simulink model "CoffeeReactor_task1"  (R2023b)
settings: Solver=ode4  StartTime=0.0  StopTime=simulationParameters.Tsim  FixedStep=simulationParameters.Tint  RelTol=1e-3
undefined symbols (not defined in the file): controller_parameters, myPID, ReactorModel_StateUpdate, simulationParameters
settings Model: Creator=simone  LastModifiedBy=viola
settings SolverCC: AlgebraicLoopSolver=TrustRegion
settings DataIOCC: SaveOutput=off  SignalLogging=off  DSMLogging=off  SaveTime=off  ReturnWorkspaceOutputs=off
settings DebuggingCC: UnconnectedInputMsg=warning  UnconnectedOutputMsg=warning  UnconnectedLineMsg=warning
settings ModelReferenceCC: EnableRefExpFcnMdlSchedulingChecks=on
settings RTWCC: DLArmComputeVersion=19.05

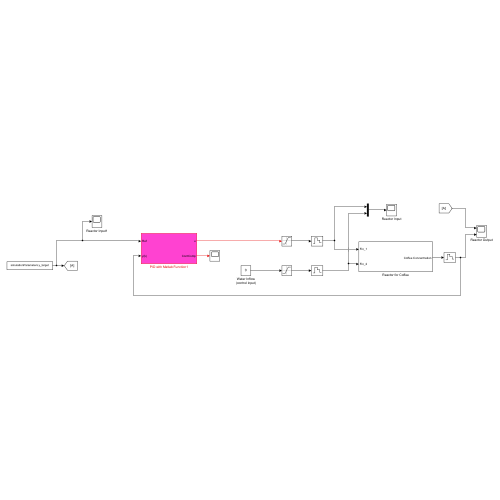
[thumbnail: Simulink's stored preview of the top-level diagram]
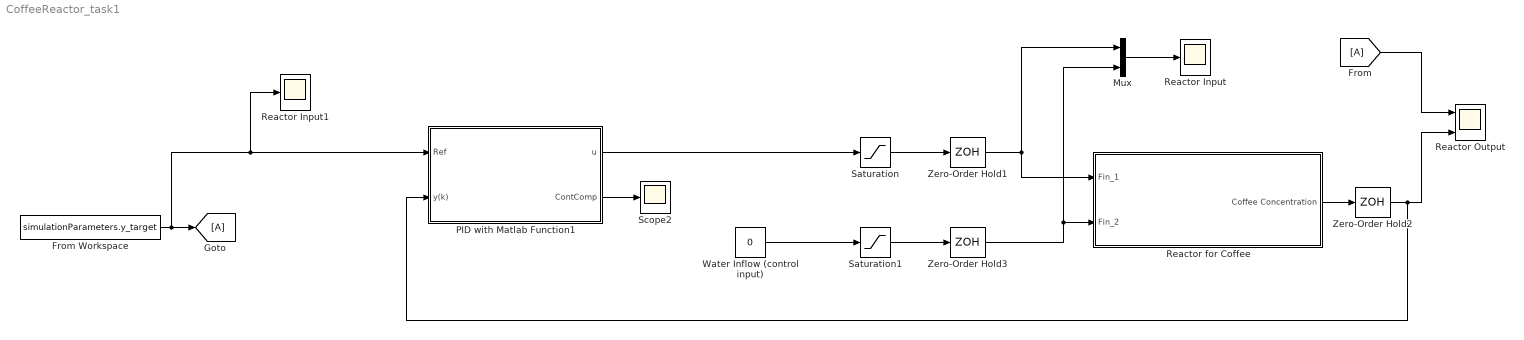
== system CoffeeReactor_task1 ==
  From : From
  From Workspace : FromWorkspace  VariableName=simulationParameters.y_target  OutputAfterFinalValue=Holding final value
  Goto : Goto
  Mux : Mux  Inputs=2
  PID with Matlab Function1 : Subsystem
  Reactor Input : Scope
  Reactor Input1 : Scope
  Reactor Output : Scope  NumInputPorts=2
  Reactor for Coffee : Subsystem
  Saturation : Saturate  UpperLimit=simulationParameters.Fin1_max  LowerLimit=simulationParameters.Fin1_min
  Saturation1 : Saturate  UpperLimit=simulationParameters.Fin2_max  LowerLimit=simulationParameters.Fin2_min
  Scope2 : Scope
  Water Inflow (control input) : Constant  Value=0
  Zero-Order Hold1 : ZeroOrderHold  SampleTime=simulationParameters.Ts
  Zero-Order Hold2 : ZeroOrderHold  SampleTime=simulationParameters.Ts
  Zero-Order Hold3 : ZeroOrderHold  SampleTime=simulationParameters.Ts
  wires:
  Reactor for Coffee/1(Coffee Concentration) -> Zero-Order Hold2/1
  Zero-Order Hold2/1 -> PID with Matlab Function1/2(y(k)), Reactor Output/2
  From/1 -> Reactor Output/1
  Mux/1 -> Reactor Input/1
  Water Inflow (control input)/1 -> Saturation1/1
  PID with Matlab Function1/1(u) -> Saturation/1
  Zero-Order Hold1/1 -> Reactor for Coffee/1(Fin_1), Mux/1
  Zero-Order Hold3/1 -> Reactor for Coffee/2(Fin_2), Mux/2
  Saturation/1 -> Zero-Order Hold1/1
  Saturation1/1 -> Zero-Order Hold3/1
  From Workspace/1 -> Reactor Input1/1, PID with Matlab Function1/1(Ref), Goto/1
  PID with Matlab Function1/2(ContComp) -> Scope2/1

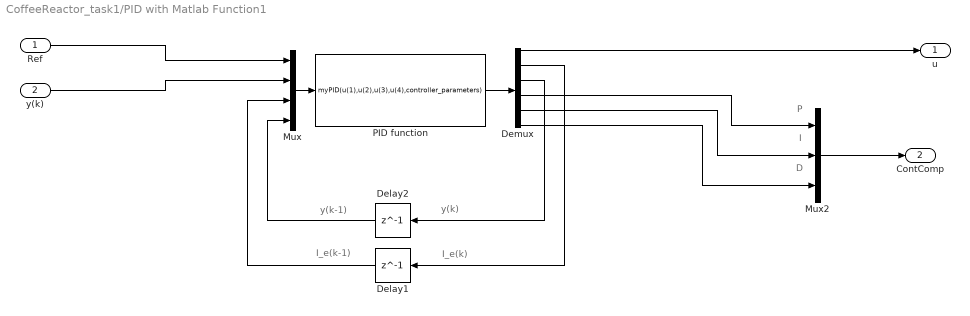
== system CoffeeReactor_task1/PID with Matlab Function1 ==
  note: y(k-1)
  note: y(k)
  note: D
  note: I
  note: P
  note: I_e(k)
  note: I_e(k-1)
  Ref : Inport
  y(k) : Inport  Port=2
  Delay1 : Delay  DelayLength=1
  Delay2 : Delay  DelayLength=1
  Demux : Demux  Outputs=6
  Mux : Mux
  Mux2 : Mux  Inputs=3
  PID function : MATLABFcn  MATLABFcn=myPID(u(1),u(2),u(3),u(4),controller_parameters)  OutputDimensions=6
  u : Outport
  ContComp : Outport  Port=2
  wires:
  Ref/1 -> Mux/1
  y(k)/1 -> Mux/2
  Mux/1 -> PID function/1
  PID function/1 -> Demux/1
  Demux/1 -> u/1
  Demux/4 -> Mux2/1
  Demux/5 -> Mux2/2
  Demux/6 -> Mux2/3
  Demux/2 -> Delay1/1
  Delay1/1 -> Mux/3
  Mux2/1 -> ContComp/1
  Delay2/1 -> Mux/4
  Demux/3 -> Delay2/1

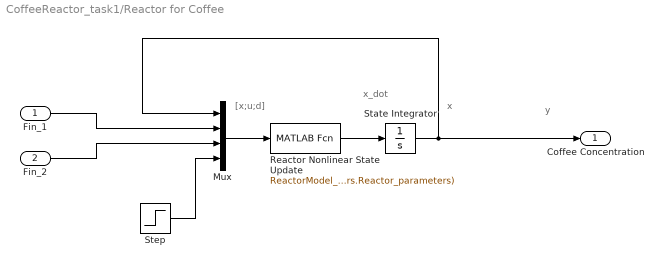
== system CoffeeReactor_task1/Reactor for Coffee ==
  note: y
  note: [x;u;d]
  note: x
  note: x_dot
  Fin_1 : Inport
  Fin_2 : Inport  Port=2
  Mux : Mux
  Reactor Nonlinear State Update : MATLABFcn  MATLABFcn=ReactorModel_StateUpdate(u(1),u(2:3),u(4),simulationParameters.Reactor_parameters)  OutputDimensions=simulationParameters.Reactor_parameters.n
  State Integrator : Integrator  InitialCondition=simulationParameters.Reactor_parameters.x_0
  Step : Step  Time=simulationParameters.Reactor_parameters.Tdist  After=simulationParameters.Reactor_parameters.Adist  SampleTime=0
  Coffee Concentration : Outport
  wires:
  Mux/1 -> Reactor Nonlinear State Update/1
  Fin_2/1 -> Mux/3
  Reactor Nonlinear State Update/1 -> State Integrator/1
  Fin_1/1 -> Mux/2
  State Integrator/1 -> Mux/1, Coffee Concentration/1
  Step/1 -> Mux/4
